simulink model "parking"  (R2021a)
settings: Solver=VariableStepAuto  StartTime=0.0  StopTime=10.0  RelTol=1e-3
libraries: fuzblock x1
settings Model: Creator=DELL  LastModifiedBy=DELL

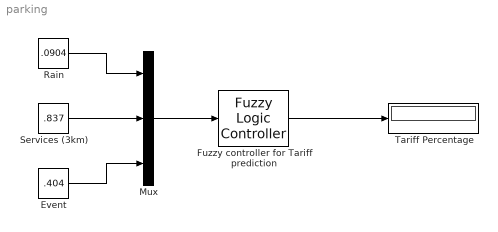
== system parking ==
  " Services (3km)" : Constant  Value=.837
  Event : Constant  Value=.404
  Fuzzy controller for Tariff prediction : fuzblock/Fuzzy Logic  Controller  FIS='ParkingTariff.fis'  OutputSampleNumber=101  DataType=double  FuzzifiedInputs=off  RuleFiringStrengths=off  RuleOutputs=off  AggregatedOutputs=off  SimulateUsing=Interpreted execution  OutOfRangeInputValueMessage=warning  NoRuleFiredMessage=warning  EmptyOutputFuzzySetMessage=warning
  Mux : Mux  Inputs=3
  Rain : Constant  Value=.0904
  Tariff Percentage : Display
  wires:
  Mux/1 -> Fuzzy controller for Tariff prediction/1
  Rain/1 -> Mux/1
  " Services (3km)"/1 -> Mux/2
  Event/1 -> Mux/3
  Fuzzy controller for Tariff prediction/1 -> Tariff Percentage/1
